simulink model "e_Aerodynamics_added"  (R2025b)
settings: Solver=ode23tb  StartTime=0.0  StopTime=20  MaxStep=0.001  RelTol=1e-3
model workspace (MAT data in the model file):
  init_r = 0
  init_vx = 0
  init_vy = 0
values from neighbouring files (symbols this model uses):
  Par =     [0_Load_data.mat]
  TireData =     [0_Load_data.mat]
libraries: simulink x3
(part 2 of 2)

== matlab function e_Aerodynamics_added/Slip Angles ==
  data: Vx input; slip_angles output; Vy input; yawrate input; Steer_FL input; Steer_FR input; Par parameter
function slip_angles = fcn(Vx, Vy, yawrate, Steer_FL, Steer_FR, Par)
%#codegen

    % 1. Geometry Setup
    L = Par.WB;
    T = Par.TW;
    
    % Distance from CG to Axles
    a = L * Par.WD_R;     
    b = L - a;             
    half_T = T / 2;

    % 2. Calculate Velocity Components at Each Corner
    % Kinematic transformation from CG to Hubs
    % Front Left (1)
        Vx_FL = Vx - yawrate * half_T;
        Vy_FL = Vy + yawrate * a;
    
    % Front Right (2)
        Vx_FR = Vx + yawrate * half_T;
        Vy_FR = Vy + yawrate * a;
    
    % Rear Left (3)
        Vx_RL = Vx - yawrate * half_T;
        Vy_RL = Vy - yawrate * b;
    
    % Rear Right (4)
        Vx_RR = Vx + yawrate * half_T;
        Vy_RR = Vy - yawrate * b;

    % 3. Calculate Velocity Angles (Theta_V)

        Theta_FL = atan2(Vy_FL, max(Vx_FL,0.1)); 
        Theta_FR = atan2(Vy_FR, max(Vx_FR,0.1));
        Theta_RL = atan2(Vy_RL, max(Vx_RL,0.1));
        Theta_RR = atan2(Vy_RR, max(Vx_RR,0.1));
    
    % 4. Construct Steering Vector (Delta)
    % Rears are assumed fixed (0 steering)
        Delta = [Steer_FL; Steer_FR; 0; 0];
    
    % Vector of Velocity Angles
        Theta_V = [Theta_FL; Theta_FR; Theta_RL; Theta_RR];

    % 5. Final Calculation
    % Alpha = Delta - Theta_V
        slip_angles = Delta - Theta_V ;
end

== matlab function e_Aerodynamics_added/Wheel to Vehicle Coordinates ==
  data: Fx_w input; Fx_b output; Fy_w input; Steer_FL input; Steer_FR input; Fy_b output; B_Fx output; B_Fy output
function [Fx_b, Fy_b, B_Fx, B_Fy] = fcn(Fx_w, Fy_w, Steer_FL, Steer_FR)
%#codegen
% FORCE & MOMENT RESOLVER
    % 1. Construct Steering Vector [FL; FR; RL; RR]
    % Rear steering is assumed to be 0
    Delta = [Steer_FL; Steer_FR; 0; 0];
    
    % 2. Pre-calculate Trig functions (Vectorized)
    c_d = cos(Delta);
    s_d = sin(Delta);
    
    % Longitudinal Body Force:

    Fx_b = Fx_w .* c_d - Fy_w .* s_d;
    
    % Lateral Body Force:
    % Fy_body = Fx_wheel * sin(delta) + Fy_wheel * cos(delta)
    Fy_b = Fx_w .* s_d + Fy_w .* c_d;
    
    % 4. Summation: Total Forces acting on CG
    B_Fx = sum(Fx_b);
    B_Fy = sum(Fy_b);
    
end

== matlab function e_Aerodynamics_added/Steering Kinematics/Steering Kinematics ==
  data: Steer_Input input; Ackermann_Pct input; Steer_FL output; Steer_FR output; Par parameter
function [Steer_FL, Steer_FR] = fcn(Steer_Input, Ackermann_Pct, Par)
%#codegen

    % 1. Constants
    L = Par.WB;      % Wheelbase
    half_T = Par.TW / 2; % Half Track Width

    % 2. Safety Clamp (Prevent tan(90) singularity)
    delta = min(max(Steer_Input, -1.5), 1.5); 
    
    % 3. Calculate "Pure Ackermann" Angles
    % Ideally, inner wheel turns sharper than outer wheel.
    tan_d = tan(delta);
    
    % FL (Left): Denom depends on sign of turn.
    % If turning Left (+), Denom shrinks (Sharper).
    FL_Ack = atan( (L * tan_d) / (L - half_T * tan_d) );
    
    % FR (Right): 
    % If turning Left (+), Denom grows (Shallower).
    FR_Ack = atan( (L * tan_d) / (L + half_T * tan_d) );
    
    % 4. Calculate "Parallel" Angles
    % Both wheels exactly match the center input
    FL_Par = delta;
    FR_Par = delta;
    
    % 5. Linear Blend based on Percentage
    % Formula: Final = Parallel + (Ackermann - Parallel) * Percent
    Steer_FL = FL_Par + (FL_Ack - FL_Par) * Ackermann_Pct;
    Steer_FR = FR_Par + (FR_Ack - FR_Par) * Ackermann_Pct;

end
